simulink model "eovsa_corr_300mhz"  (R2012b)
settings: Solver=VariableStepDiscrete  SolverMode=SingleTasking  StartTime=0.0  StopTime=5000  RelTol=1e-3
undefined symbols (not defined in the file or in its folder): A, B, gcbh, PCIN, sfp, xlBlockLoadCallback, xlipgetpartsetting
libraries: xbsIndex_r4 x5996, casper_library_misc x52, simulink x33, dspsigops x24, xps_library x15, casper_library_delays x2
(part 26 of 65)

== system eovsa_corr_300mhz/vector_acc/power_sq_acc ==
  note: There is a bug in this green block.
      | Its output is held high for veector length number of pulses initially event without new_acc pulse.
  sync : Inport
  acc_length : Inport  Port=2
  sq_power_in0 : Inport  Port=3
  sq_power_in1 : Inport  Port=4
  sq_power_in2 : Inport  Port=5
  sq_power_in3 : Inport  Port=6
  sq_power_in4 : Inport  Port=7
  sq_power_in5 : Inport  Port=8
  sq_power_in6 : Inport  Port=9
  sq_power_in7 : Inport  Port=10
  acc_start_skip : Inport  Port=11
  Delay{1,3,6,9,14,17,21,24..40} (24 alike) : xbsIndex_r4/Delay  rst=off  infoeditControl=Selection of Reset will increase slice count due to use of real FFs and instead of SRLs  en=off  latency=1  dbl_ovrd=off  reg_retiming=on  block_type=delay
      settings: block_version=11.4
  Delay{2,4..5,7..8,10..13,15..16,18..20,22..23,41..42} (18 alike) : xbsIndex_r4/Delay  rst=off  infoeditControl=Selection of Reset will increase slice count due to use of real FFs and instead of SRLs  en=off  latency=1  dbl_ovrd=off  reg_retiming=off  block_type=delay
      settings: block_version=11.4
  Terminator{1..6,24} (7 alike) : Terminator
  new_acc1 : Subsystem
  wide_bram_vacc : Subsystem  AncestorBlock=casper_library_accumulators/wide_bram_vacc  mask(wide_bram_vacc){vec_len=2048, arith_type=Unsigned, n_bits=64, bin_pt=44}
      mask prompts: vec_len "Vector length:"; arith_type "Arithmetic type (input/output):"; n_bits "Bit width (output):"; bin_pt "Binary point (output):"
      mask help:
      | This vector accumulator based on DSP48 slices and BRAMs is designed for wide accumulators (48 < output width <= 96).
      |
      | It outputs its previous accumulated vector after a new_acc pulse is received.
      |
      | The "Data IN" (din) value is used if "Data OK" (dok) is 1, otherwise a 0 value is accumulated instead.  This can be used, for example, to implement blanking without requiring external multiplexers.
      mask init:
      | set_param([gcb,'/outsize/Reinterpret'], 'arith_type', arith_type);
      mask TypeOptions arith_type: Signed  (2's comp) | Unsigned
  wide_bram_vacc1 : Subsystem  AncestorBlock=casper_library_accumulators/wide_bram_vacc  mask(wide_bram_vacc){vec_len=2048, arith_type=Unsigned, n_bits=64, bin_pt=44}
      mask prompts: vec_len "Vector length:"; arith_type "Arithmetic type (input/output):"; n_bits "Bit width (output):"; bin_pt "Binary point (output):"
      mask help:
      | This vector accumulator based on DSP48 slices and BRAMs is designed for wide accumulators (48 < output width <= 96).
      |
      | It outputs its previous accumulated vector after a new_acc pulse is received.
      |
      | The "Data IN" (din) value is used if "Data OK" (dok) is 1, otherwise a 0 value is accumulated instead.  This can be used, for example, to implement blanking without requiring external multiplexers.
      mask init:
      | set_param([gcb,'/outsize/Reinterpret'], 'arith_type', arith_type);
      mask TypeOptions arith_type: Signed  (2's comp) | Unsigned
  wide_bram_vacc2 : Subsystem  AncestorBlock=casper_library_accumulators/wide_bram_vacc  mask(wide_bram_vacc){vec_len=2048, arith_type=Unsigned, n_bits=64, bin_pt=44}
      mask prompts: vec_len "Vector length:"; arith_type "Arithmetic type (input/output):"; n_bits "Bit width (output):"; bin_pt "Binary point (output):"
      mask help:
      | This vector accumulator based on DSP48 slices and BRAMs is designed for wide accumulators (48 < output width <= 96).
      |
      | It outputs its previous accumulated vector after a new_acc pulse is received.
      |
      | The "Data IN" (din) value is used if "Data OK" (dok) is 1, otherwise a 0 value is accumulated instead.  This can be used, for example, to implement blanking without requiring external multiplexers.
      mask init:
      | set_param([gcb,'/outsize/Reinterpret'], 'arith_type', arith_type);
      mask TypeOptions arith_type: Signed  (2's comp) | Unsigned
  wide_bram_vacc3 : Subsystem  AncestorBlock=casper_library_accumulators/wide_bram_vacc  mask(wide_bram_vacc){vec_len=2048, arith_type=Unsigned, n_bits=64, bin_pt=44}
      mask prompts: vec_len "Vector length:"; arith_type "Arithmetic type (input/output):"; n_bits "Bit width (output):"; bin_pt "Binary point (output):"
      mask help:
      | This vector accumulator based on DSP48 slices and BRAMs is designed for wide accumulators (48 < output width <= 96).
      |
      | It outputs its previous accumulated vector after a new_acc pulse is received.
      |
      | The "Data IN" (din) value is used if "Data OK" (dok) is 1, otherwise a 0 value is accumulated instead.  This can be used, for example, to implement blanking without requiring external multiplexers.
      mask init:
      | set_param([gcb,'/outsize/Reinterpret'], 'arith_type', arith_type);
      mask TypeOptions arith_type: Signed  (2's comp) | Unsigned
  wide_bram_vacc4 : Subsystem  AncestorBlock=casper_library_accumulators/wide_bram_vacc  mask(wide_bram_vacc){vec_len=2048, arith_type=Unsigned, n_bits=64, bin_pt=44}
      mask prompts: vec_len "Vector length:"; arith_type "Arithmetic type (input/output):"; n_bits "Bit width (output):"; bin_pt "Binary point (output):"
      mask help:
      | This vector accumulator based on DSP48 slices and BRAMs is designed for wide accumulators (48 < output width <= 96).
      |
      | It outputs its previous accumulated vector after a new_acc pulse is received.
      |
      | The "Data IN" (din) value is used if "Data OK" (dok) is 1, otherwise a 0 value is accumulated instead.  This can be used, for example, to implement blanking without requiring external multiplexers.
      mask init:
      | set_param([gcb,'/outsize/Reinterpret'], 'arith_type', arith_type);
      mask TypeOptions arith_type: Signed  (2's comp) | Unsigned
  wide_bram_vacc5 : Subsystem  AncestorBlock=casper_library_accumulators/wide_bram_vacc  mask(wide_bram_vacc){vec_len=2048, arith_type=Unsigned, n_bits=64, bin_pt=44}
      mask prompts: vec_len "Vector length:"; arith_type "Arithmetic type (input/output):"; n_bits "Bit width (output):"; bin_pt "Binary point (output):"
      mask help:
      | This vector accumulator based on DSP48 slices and BRAMs is designed for wide accumulators (48 < output width <= 96).
      |
      | It outputs its previous accumulated vector after a new_acc pulse is received.
      |
      | The "Data IN" (din) value is used if "Data OK" (dok) is 1, otherwise a 0 value is accumulated instead.  This can be used, for example, to implement blanking without requiring external multiplexers.
      mask init:
      | set_param([gcb,'/outsize/Reinterpret'], 'arith_type', arith_type);
      mask TypeOptions arith_type: Signed  (2's comp) | Unsigned
  wide_bram_vacc6 : Subsystem  AncestorBlock=casper_library_accumulators/wide_bram_vacc  mask(wide_bram_vacc){vec_len=2048, arith_type=Unsigned, n_bits=64, bin_pt=44}
      mask prompts: vec_len "Vector length:"; arith_type "Arithmetic type (input/output):"; n_bits "Bit width (output):"; bin_pt "Binary point (output):"
      mask help:
      | This vector accumulator based on DSP48 slices and BRAMs is designed for wide accumulators (48 < output width <= 96).
      |
      | It outputs its previous accumulated vector after a new_acc pulse is received.
      |
      | The "Data IN" (din) value is used if "Data OK" (dok) is 1, otherwise a 0 value is accumulated instead.  This can be used, for example, to implement blanking without requiring external multiplexers.
      mask init:
      | set_param([gcb,'/outsize/Reinterpret'], 'arith_type', arith_type);
      mask TypeOptions arith_type: Signed  (2's comp) | Unsigned
  wide_bram_vacc7 : Subsystem  AncestorBlock=casper_library_accumulators/wide_bram_vacc  mask(wide_bram_vacc){vec_len=2048, arith_type=Unsigned, n_bits=64, bin_pt=44}
      mask prompts: vec_len "Vector length:"; arith_type "Arithmetic type (input/output):"; n_bits "Bit width (output):"; bin_pt "Binary point (output):"
      mask help:
      | This vector accumulator based on DSP48 slices and BRAMs is designed for wide accumulators (48 < output width <= 96).
      |
      | It outputs its previous accumulated vector after a new_acc pulse is received.
      |
      | The "Data IN" (din) value is used if "Data OK" (dok) is 1, otherwise a 0 value is accumulated instead.  This can be used, for example, to implement blanking without requiring external multiplexers.
      mask init:
      | set_param([gcb,'/outsize/Reinterpret'], 'arith_type', arith_type);
      mask TypeOptions arith_type: Signed  (2's comp) | Unsigned
  data_valid : Outport
  power_sq0 : Outport  Port=2
  power_sq1 : Outport  Port=3
  power_sq2 : Outport  Port=4
  power_sq3 : Outport  Port=5
  power_sq4 : Outport  Port=6
  power_sq5 : Outport  Port=7
  power_sq6 : Outport  Port=8
  power_sq7 : Outport  Port=9
  wires:
  wide_bram_vacc/2(valid) -> data_valid/1
  wide_bram_vacc/1(dout) -> power_sq0/1
  wide_bram_vacc1/1(dout) -> power_sq1/1
  sync/1 -> new_acc1/1(sync)
  wide_bram_vacc1/2(valid) -> Terminator24/1
  wide_bram_vacc2/2(valid) -> Terminator1/1
  wide_bram_vacc2/1(dout) -> power_sq2/1
  wide_bram_vacc3/1(dout) -> power_sq3/1
  wide_bram_vacc4/2(valid) -> Terminator2/1
  wide_bram_vacc4/1(dout) -> power_sq4/1
  wide_bram_vacc5/2(valid) -> Terminator4/1
  wide_bram_vacc5/1(dout) -> power_sq5/1
  wide_bram_vacc6/1(dout) -> power_sq6/1
  wide_bram_vacc6/2(valid) -> Terminator6/1
  acc_length/1 -> new_acc1/2(acc_len)
  acc_start_skip/1 -> new_acc1/3(acc_start_skip)
  new_acc1/2(use_data) -> Delay41/1
  [use_data] -> Delay2/1
  new_acc1/1(new_acc) -> Delay42/1
  [new_acc] -> Delay19/1
  [use_data] -> Delay5/1
  [new_acc] -> Delay4/1
  [use_data] -> Delay8/1
  [new_acc] -> Delay7/1
  [use_data] -> Delay11/1
  [new_acc] -> Delay10/1
  [use_data] -> Delay13/1
  [new_acc] -> Delay12/1
  [use_data] -> Delay16/1
  [new_acc] -> Delay15/1
  [use_data] -> Delay20/1
  [new_acc] -> Delay18/1
  [use_data] -> Delay23/1
  [new_acc] -> Delay22/1
  sq_power_in0/1 -> Delay25/1
  sq_power_in1/1 -> Delay26/1
  sq_power_in2/1 -> Delay27/1
  sq_power_in3/1 -> Delay28/1
  sq_power_in4/1 -> Delay29/1
  sq_power_in5/1 -> Delay30/1
  sq_power_in7/1 -> Delay32/1
  sq_power_in6/1 -> Delay31/1
  Delay1/1 -> wide_bram_vacc/2(din)
  Delay2/1 -> wide_bram_vacc/3(dok)
  Delay19/1 -> wide_bram_vacc/1(new_acc)
  Delay3/1 -> wide_bram_vacc1/2(din)
  Delay4/1 -> wide_bram_vacc1/1(new_acc)
  Delay5/1 -> wide_bram_vacc1/3(dok)
  Delay6/1 -> wide_bram_vacc2/2(din)
  Delay7/1 -> wide_bram_vacc2/1(new_acc)
  Delay8/1 -> wide_bram_vacc2/3(dok)
  Delay10/1 -> wide_bram_vacc3/1(new_acc)
  Delay9/1 -> wide_bram_vacc3/2(din)
  Delay11/1 -> wide_bram_vacc3/3(dok)
  Delay14/1 -> wide_bram_vacc4/2(din)
  Delay13/1 -> wide_bram_vacc4/3(dok)
  Delay12/1 -> wide_bram_vacc4/1(new_acc)
  Delay16/1 -> wide_bram_vacc5/3(dok)
  Delay15/1 -> wide_bram_vacc5/1(new_acc)
  Delay17/1 -> wide_bram_vacc5/2(din)
  Delay18/1 -> wide_bram_vacc6/1(new_acc)
  Delay20/1 -> wide_bram_vacc6/3(dok)
  Delay21/1 -> wide_bram_vacc6/2(din)
  Delay25/1 -> Delay33/1
  Delay26/1 -> Delay34/1
  Delay27/1 -> Delay35/1
  Delay28/1 -> Delay36/1
  Delay29/1 -> Delay37/1
  Delay30/1 -> Delay38/1
  Delay31/1 -> Delay39/1
  Delay32/1 -> Delay40/1
  Delay33/1 -> Delay1/1
  Delay34/1 -> Delay3/1
  Delay35/1 -> Delay6/1
  Delay36/1 -> Delay9/1
  Delay37/1 -> Delay14/1
  Delay38/1 -> Delay17/1
  Delay39/1 -> Delay21/1
  Delay40/1 -> Delay24/1
  Delay41/1 -> [use_data]
  Delay42/1 -> [new_acc]
  wide_bram_vacc3/2(valid) -> Terminator3/1
  Delay23/1 -> wide_bram_vacc7/3(dok)
  Delay24/1 -> wide_bram_vacc7/2(din)
  Delay22/1 -> wide_bram_vacc7/1(new_acc)
  wide_bram_vacc7/1(dout) -> power_sq7/1
  wide_bram_vacc7/2(valid) -> Terminator5/1

== system eovsa_corr_300mhz/xeng0_vacc/edge_detect ==
  in : Inport
  Delay : xbsIndex_r4/Delay  rst=off  infoeditControl=Selection of Reset will increase slice count due to use of real FFs and instead of SRLs  en=off  latency=1  dbl_ovrd=off  reg_retiming=on  block_type=delay
      settings: xl_area=[0, 0, 0, 0, 0, 0, 0]
  Inverter : xbsIndex_r4/Inverter  en=off  latency=0  dbl_ovrd=off  block_type=inv
      settings: xl_area=[0, 0, 0, 0, 0, 0, 0]
  edge_op : xbsIndex_r4/Logical  logical_function=NOR  inputs=2  en=off  latency=0  precision=Full  arith_type=Unsigned  n_bits=8  bin_pt=2  align_bp=on  dbl_ovrd=off  block_type=logical
      settings: xl_area=[0, 0, 0, 0, 0, 0, 0]
  out : Outport
  wires:
  Inverter/1 -> edge_op/1
  edge_op/1 -> out/1
  in/1 -> Inverter/1, Delay/1
  Delay/1 -> edge_op/2

== system eovsa_corr_300mhz/xeng0_vacc/qv1 ==
  note: Compensate for the latency
      | of the vacc controller here.
      | (it sets rd_en high a clock
      | after vld goes high)
      | Then it takes a further clock to
      | mux and register the addr / enable signals
  rst : Inport
  rb_burst_len_mi : Inport  Port=2
  vld : Inport  Port=3
  sync : Inport  Port=4
  acc_len_mi : Inport  Port=5
  din : Inport  Port=6
  Constant : xbsIndex_r4/Constant  const="2^8 -  1"  gui_display_data_type=Fixed-point  arith_type=Unsigned  n_bits=8  bin_pt=0  preci_type=Single  exp_width=8  frac_width=24  explicit_period=on  period=1  equ=P=C  opselect=C  inp2=PCIN>>17  opr=+  inp1=P  carry=CIN  dbl_ovrd=off  block_type=constant
  Delay1 : xbsIndex_r4/Delay  rst=off  infoeditControl=Selection of Reset will increase slice count due to use of real FFs and instead of SRLs  en=off  latency=12-1  dbl_ovrd=off  reg_retiming=on  block_type=delay
  Delay2 : xbsIndex_r4/Delay  rst=off  infoeditControl=Selection of Reset will increase slice count due to use of real FFs and instead of SRLs  en=off  latency=2  dbl_ovrd=off  reg_retiming=on  block_type=delay
  Delay3 : xbsIndex_r4/Delay  rst=off  infoeditControl=Selection of Reset will increase slice count due to use of real FFs and instead of SRLs  en=off  latency=1  dbl_ovrd=off  reg_retiming=off  block_type=delay
  Delay4 : xbsIndex_r4/Delay  rst=off  infoeditControl=Selection of Reset will increase slice count due to use of real FFs and instead of SRLs  en=off  latency=2  dbl_ovrd=off  reg_retiming=off  block_type=delay
  Delay5 : xbsIndex_r4/Delay  rst=off  infoeditControl=Selection of Reset will increase slice count due to use of real FFs and instead of SRLs  en=off  latency=1  dbl_ovrd=off  reg_retiming=off  block_type=delay
  Delay6 : xbsIndex_r4/Delay  rst=off  infoeditControl=Selection of Reset will increase slice count due to use of real FFs and instead of SRLs  en=off  latency=12-1  dbl_ovrd=off  reg_retiming=on  block_type=delay
  Gateway Out{1..8} (8 alike) : xbsIndex_r4/Gateway Out  inherit_from_input=off  hdl_port=on  timing_constraint=None  locs_specified=off  LOCs={}  UseAsDAC=off  DACChannel='1'  block_type=gatewayout
  Inverter : xbsIndex_r4/Inverter  en=off  latency=0  dbl_ovrd=off  block_type=inv
  Inverter1 : xbsIndex_r4/Inverter  en=off  latency=0  dbl_ovrd=off  block_type=inv
  Logical : xbsIndex_r4/Logical  logical_function=AND  inputs=2  en=off  latency=0  precision=Full  arith_type=Unsigned  n_bits=16  bin_pt=0  align_bp=on  dbl_ovrd=off  block_type=logical
  Logical1 : xbsIndex_r4/Logical  logical_function=AND  inputs=2  en=off  latency=0  precision=Full  arith_type=Unsigned  n_bits=16  bin_pt=0  align_bp=on  dbl_ovrd=off  block_type=logical
  Scope : Scope  NumInputPorts=8
      settings: YMin=-5~-5~-5~-5~-5~-5~-5~-5  YMax=5~5~5~5~5~5~5~5
  Slice4 : xbsIndex_r4/Slice  nbits=64  boolean_output=off  mode=Lower Bit Location + Width  bit1=0  base1=MSB of Input  bit0=0  base0=LSB of Input  dbl_ovrd=off  block_type=slice
  Slice_A : xbsIndex_r4/Slice  nbits=32  boolean_output=off  mode=Lower Bit Location + Width  bit1=0  base1=MSB of Input  bit0=32  base0=LSB of Input  dbl_ovrd=off  block_type=slice
  Slice_A1 : xbsIndex_r4/Slice  nbits=32  boolean_output=off  mode=Lower Bit Location + Width  bit1=0  base1=MSB of Input  bit0=32  base0=LSB of Input  dbl_ovrd=off  block_type=slice
  Slice_A2 : xbsIndex_r4/Slice  nbits=32  boolean_output=off  mode=Lower Bit Location + Width  bit1=0  base1=MSB of Input  bit0=0  base0=LSB of Input  dbl_ovrd=off  block_type=slice
  Slice_A3 : xbsIndex_r4/Slice  nbits=32  boolean_output=off  mode=Lower Bit Location + Width  bit1=0  base1=MSB of Input  bit0=0  base0=LSB of Input  dbl_ovrd=off  block_type=slice
  adder1 : Subsystem
  adder2 : Subsystem
  bus_create : Subsystem  AncestorBlock=casper_library_flow_control/bus_create  mask(bus_create){inputNum=2}
      mask prompts: inputNum "Number of inputs:"
      mask init:
      | bus_create_init(gcb,...
      |     'inputNum', inputNum);
  pipeline1 : Subsystem  AncestorBlock=casper_library_delays/pipeline  mask(pipeline){latency=1}
      mask help:
      | An explicitly laid-out delay line to avoid mapping to SRL16s
      | for use in pipelining to help achieve timing closure.
      mask init:
      | pipeline_init(gcb,'latency',latency);
      settings: AttributesFormatString=Latency = %<latency>
      mask Display:
      | port_label('input', 1, 'd');
      | port_label('output', 1, 'q');
      | disp(['Z^-', num2str(latency)]);
  pipeline2 : Subsystem  AncestorBlock=casper_library_delays/pipeline  mask(pipeline){latency=1}
      mask help:
      | An explicitly laid-out delay line to avoid mapping to SRL16s
      | for use in pipelining to help achieve timing closure.
      mask init:
      | pipeline_init(gcb,'latency',latency);
      settings: AttributesFormatString=Latency = %<latency>
      mask Display:
      | port_label('input', 1, 'd');
      | port_label('output', 1, 'q');
      | disp(['Z^-', num2str(latency)]);
  pipeline3 : Subsystem  AncestorBlock=casper_library_delays/pipeline  mask(pipeline){latency=1}
      mask help:
      | An explicitly laid-out delay line to avoid mapping to SRL16s
      | for use in pipelining to help achieve timing closure.
      mask init:
      | pipeline_init(gcb,'latency',latency);
      settings: AttributesFormatString=Latency = %<latency>
      mask Display:
      | port_label('input', 1, 'd');
      | port_label('output', 1, 'q');
      | disp(['Z^-', num2str(latency)]);
  pipeline5 : Subsystem  AncestorBlock=casper_library_delays/pipeline  mask(pipeline){latency=1}
      mask help:
      | An explicitly laid-out delay line to avoid mapping to SRL16s
      | for use in pipelining to help achieve timing closure.
      mask init:
      | pipeline_init(gcb,'latency',latency);
      settings: AttributesFormatString=Latency = %<latency>
      mask Display:
      | port_label('input', 1, 'd');
      | port_label('output', 1, 'q');
      | disp(['Z^-', num2str(latency)]);
  pipeline6 : Subsystem  AncestorBlock=casper_library_delays/pipeline  mask(pipeline){latency=1}
      mask help:
      | An explicitly laid-out delay line to avoid mapping to SRL16s
      | for use in pipelining to help achieve timing closure.
      mask init:
      | pipeline_init(gcb,'latency',latency);
      settings: AttributesFormatString=Latency = %<latency>
      mask Display:
      | port_label('input', 1, 'd');
      | port_label('output', 1, 'q');
      | disp(['Z^-', num2str(latency)]);
  pipeline93 : Subsystem  AncestorBlock=casper_library_delays/pipeline  mask(pipeline){latency=1}
      mask help:
      | An explicitly laid-out delay line to avoid mapping to SRL16s
      | for use in pipelining to help achieve timing closure.
      mask init:
      | pipeline_init(gcb,'latency',latency);
      settings: AttributesFormatString=Latency = %<latency>
      mask Display:
      | port_label('input', 1, 'd');
      | port_label('output', 1, 'q');
      | disp(['Z^-', num2str(latency)]);
  qdr : xps_library/qdr  Tag=xps:qdr  which_qdr=qdr0  qdr_awidth=12  use_sniffer=on
  qdr_vacc_ctrl : Subsystem  mask{qdr_latency=12, add_latency=3, vec_len=vector_len}
      mask prompts: qdr_latency "QDR Latency?"; add_latency "Add latency?"; vec_len "Vector length?"
  dout : Outport
  dout_vld : Outport  Port=2
  first_vec : Outport  Port=3
  wires:
  Constant/1 -> qdr/3
  qdr/1 -> Slice4/1
  din/1 -> Delay2/1
  Delay1/1 -> pipeline1/1(d)
  [qdr_dout] -> Slice_A2/1  "adder_mem_in"
  pipeline1/1(q) -> Slice_A3/1  "adder_din"
  Slice4/1 -> pipeline5/1(d)
  [qdr_dout] -> dout/1  "vacc_dout"
  [rb_vld] -> dout_vld/1  "vacc_dvld"
  pipeline3/1(q) -> qdr/4  "adr_addr"
  Delay4/1 -> Delay5/1  "qdr_din"
  pipeline5/1(q) -> [qdr_dout]  "vacc_dout"
  bus_create/1(bus_out) -> Delay3/1
  Delay2/1 -> Delay6/1, Delay1/1
  [first_vec] -> adder1/3(new_acc)  "adder_first_vec"
  Delay3/1 -> Delay4/1
  [first_vec] -> first_vec/1
  rst/1 -> Gateway Out8/1, Inverter1/1, Inverter/1, qdr_vacc_ctrl/1(rst)  "rst"
  rb_burst_len_mi/1 -> Gateway Out1/1, qdr_vacc_ctrl/2(rb_burst_len_mi)  "burst length"
  vld/1 -> Gateway Out2/1, qdr_vacc_ctrl/3(vld)  "vld"
  sync/1 -> Gateway Out3/1, qdr_vacc_ctrl/4(sync)  "sync"
  acc_len_mi/1 -> Gateway Out7/1, qdr_vacc_ctrl/5(acc_len_mi)  "acc len"
  qdr_vacc_ctrl/1(qdr_re) -> Logical/2, Gateway Out4/1
  qdr_vacc_ctrl/2(qdr_we) -> Logical1/2, Gateway Out5/1
  qdr_vacc_ctrl/3(qdr_addr) -> Gateway Out6/1, pipeline3/1(d)
  qdr_vacc_ctrl/4(dout_vld) -> [rb_vld]
  qdr_vacc_ctrl/5(final_vec) -> [first_vec]
  Gateway Out2/1 -> Scope/3
  Gateway Out8/1 -> Scope/1
  Gateway Out7/1 -> Scope/5
  Gateway Out3/1 -> Scope/4
  Gateway Out6/1 -> Scope/8
  Gateway Out1/1 -> Scope/2
  Gateway Out5/1 -> Scope/7
  Gateway Out4/1 -> Scope/6
  Inverter/1 -> Logical/1
  pipeline2/1(q) -> qdr/2  "qdr_wr_en"
  pipeline93/1(q) -> qdr/1  "qdr_rd_en"
  Logical/1 -> pipeline93/1(d)
  Inverter1/1 -> Logical1/1
  Logical1/1 -> pipeline2/1(d)
  [first_vec] -> adder2/3(new_acc)
  Delay6/1 -> pipeline6/1(d)
  pipeline6/1(q) -> Slice_A1/1
  [qdr_dout] -> Slice_A/1
  Slice_A/1 -> adder2/1(buf_in)
  Slice_A1/1 -> adder2/2(din)
  Slice_A2/1 -> adder1/1(buf_in)
  Slice_A3/1 -> adder1/2(din)
  adder2/1(out) -> bus_create/1(in1)
  adder1/1(out) -> bus_create/2(in2)  "adder_dout"
  Delay5/1 -> qdr/5

== system eovsa_corr_300mhz/xeng_hdl_uint/xeng_descramble ==
  note: x_cast is necessary to correct for BRAM
      | readout order
  note: This bit of logic
      | ensures that we only send out
      | a sync if one was received
      | (and then align it with the start of a read)
  acc : Inport
  valid : Inport  Port=2
  sync : Inport  Port=3
  win_valid : Inport  Port=4
  Constant2 : xbsIndex_r4/Constant  const=0  gui_display_data_type=Fixed-point  arith_type=Boolean  n_bits=elements_bits + 1  bin_pt=0  preci_type=Single  exp_width=8  frac_width=24  explicit_period=on  period=1  equ=P=C  opselect=C  inp2=PCIN>>17  opr=+  inp1=P  carry=CIN  dbl_ovrd=off  block_type=constant
      settings: block_version=9.2.01
  Constant3 : xbsIndex_r4/Constant  const=0  gui_display_data_type=Fixed-point  arith_type=Unsigned  n_bits=n_bits_in/demux_factor  bin_pt=0  preci_type=Single  exp_width=8  frac_width=24  explicit_period=on  period=1  equ=P=C  opselect=C  inp2=PCIN>>17  opr=+  inp1=P  carry=CIN  dbl_ovrd=off  block_type=constant
      settings: block_version=9.2.01
  Delay1 : xbsIndex_r4/Delay  rst=off  infoeditControl=Selection of Reset will increase slice count due to use of real FFs and instead of SRLs  en=off  latency=3  dbl_ovrd=off  reg_retiming=off  block_type=delay
      settings: xl_area=[0, 0, 0, 0, 0, 0, 0]  block_version=9.2.01
  Delay{2..4,7} (4 alike) : xbsIndex_r4/Delay  rst=off  infoeditControl=Selection of Reset will increase slice count due to use of real FFs and instead of SRLs  en=off  latency=1  dbl_ovrd=off  reg_retiming=off  block_type=delay
      settings: xl_area=[0, 0, 0, 0, 0, 0, 0]  block_version=9.2.01
  Delay5 : xbsIndex_r4/Delay  rst=off  infoeditControl=Selection of Reset will increase slice count due to use of real FFs and instead of SRLs  en=off  latency=2  dbl_ovrd=off  reg_retiming=off  block_type=delay
      settings: xl_area=[0, 0, 0, 0, 0, 0, 0]  block_version=9.2.01
  Delay6 : xbsIndex_r4/Delay  rst=off  infoeditControl=Selection of Reset will increase slice count due to use of real FFs and instead of SRLs  en=off  latency=2  dbl_ovrd=off  reg_retiming=off  block_type=delay
      settings: xl_area=[0, 0, 0, 0, 0, 0, 0]  block_version=9.2.01
  Dual Port RAM : xbsIndex_r4/Dual Port RAM  depth=(num_elements+1)*demux_factor  initVector=[1:36*8]  distributed_mem=Block RAM  init_a=0  init_b=0  rst_a=off  rst_b=off  en_a=off  en_b=off  latency=3  write_mode_A=No Read On Write  write_mode_B=No Read On Write  dbl_ovrd=off  optimize=Speed  block_type=dpram
      settings: xl_area=[0, 0, 0, 0, 0, 0, 0]  block_version=9.2.01
  Gateway Out{4..11} (8 alike) : xbsIndex_r4/Gateway Out  inherit_from_input=off  hdl_port=off  timing_constraint=None  locs_specified=off  LOCs={}  UseAsDAC=off  DACChannel='1'  block_type=gatewayout
      settings: infoedit="Gateway out block.  Converts Xilinx fixed point inputs into ouputs of type Simulink integer, double, or fixed point.<P><P>Hardware notes:  In hardware these blocks become top level output ports or are discarded, depending on how they are configured."  xl_area=[0 0 0 0 0 0 0]  block_version=10.1.3
  Logical : xbsIndex_r4/Logical  logical_function=AND  inputs=2  en=off  latency=3  precision=Full  arith_type=Unsigned  n_bits=16  bin_pt=0  align_bp=on  dbl_ovrd=off  block_type=logical
  Register : xbsIndex_r4/Register  init=0  rst=on  en=on  dbl_ovrd=off  block_type=register
  Scope1 : Scope  NumInputPorts=8
      settings: TimeRange=70000  YMin=0~0~0~0~0~0~0~0  YMax=1~1~1~1~1~35~1~35  SaveName=ScopeData3
  Terminator1 : Terminator
  read_ctrl : Subsystem  AncestorBlock=casper_library_correlator/xeng_mask/win2_ctrl
  write_ctrl : Subsystem  AncestorBlock=casper_library_correlator/xeng_mask/win2_ctrl
  x_cast : Subsystem  AncestorBlock=casper_library_correlator/x_cast  mask{n_bits_in=n_bits_xeng_out, n_bits_out=n_bits_in/8, fix_pnt_pos=(n_bits-1)*2, demux_factor=demux_factor}
      mask prompts: n_bits_in "Number of bits (input)"; n_bits_out "Number of bits (output)"; fix_pnt_pos "Fixed point position"; demux_factor "Demux Factor"
      mask init:
      | switch (demux_factor)
      |     case (8)
      |         bit_offsets=[0 1 2 3 4 5 6 7];
      |     case (4) 
      |         bit_offsets=[1 0 3 2 5 4 7 6];  
      |     case (2) 
      |         bit_offsets=[3 2 1 0 7 6 5 4];  
      |     case (1) 
      |         bit_offsets=[7 6 5 4 3 2 1 0];  
      | end
      | 
      | 
      | fmtstr = sprintf('%d -> %d, demux %d.',n_bits_in,n_bits_out,demux_factor);
      | set_param(gcb, 'AttributesFormatString', fmtstr);
      settings: AttributesFormatString=18 -> 32, demux 4.
  acc_out : Outport
  valid_out : Outport  Port=2
  sync_out : Outport  Port=3
  wires:
  x_cast/1(out) -> Delay3/1
  Delay6/1 -> Gateway Out6/1
  Delay5/1 -> Gateway Out8/1
  [sync_in] -> Register/3
  [sync_in] -> Register/1
  [sync_in] -> Gateway Out5/1
  [valid_out] -> Gateway Out7/1
  [valid_out] -> Delay1/1
  read_ctrl/2(enable) -> [valid_out]
  [start_read] -> Gateway Out4/1
  [start_read] -> Register/2
  [start_read] -> Logical/1
  [start_read] -> read_ctrl/1(start)
  write_ctrl/1(start_readout) -> [start_read]
  win_valid/1 -> Delay5/1, write_ctrl/4(window_valid)
  Register/1 -> Logical/2
  Logical/1 -> sync_out/1
  Gateway Out10/1 -> Scope1/7
  Gateway Out9/1 -> Scope1/6
  Gateway Out7/1 -> Scope1/5
  Gateway Out4/1 -> Scope1/4
  Gateway Out5/1 -> Scope1/1
  Gateway Out6/1 -> Scope1/2
  Gateway Out8/1 -> Scope1/3
  Dual Port RAM/2 -> Terminator1/1
  acc/1 -> write_ctrl/2(data_in)
  write_ctrl/3(data_out) -> x_cast/1(in)
  Constant3/1 -> Dual Port RAM/2
  write_ctrl/4(enable) -> Delay2/1, Gateway Out10/1
  Constant2/1 -> Dual Port RAM/3
  Delay1/1 -> valid_out/1
  Dual Port RAM/1 -> acc_out/1
  read_ctrl/1(read_addr) -> Gateway Out9/1, Delay7/1
  write_ctrl/2(write_addr) -> Delay4/1, Gateway Out11/1
  sync/1 -> [sync_in], write_ctrl/1(sync)
  valid/1 -> Delay6/1, write_ctrl/3(xeng_valid)
  Gateway Out11/1 -> Scope1/8
  Delay2/1 -> Dual Port RAM/6
  Delay3/1 -> Dual Port RAM/5
  Delay4/1 -> Dual Port RAM/4
  Delay7/1 -> Dual Port RAM/1

== system eovsa_corr_300mhz/acc_sync/gen_N_pps/edge_detect2 ==
  in : Inport
  Delay : xbsIndex_r4/Delay  rst=off  infoeditControl=Selection of Reset will increase slice count due to use of real FFs and instead of SRLs  en=off  latency=1  dbl_ovrd=off  reg_retiming=on  block_type=delay
      settings: xl_area=[0, 0, 0, 0, 0, 0, 0]
  Inverter : xbsIndex_r4/Inverter  en=off  latency=0  dbl_ovrd=off  block_type=inv
      settings: xl_area=[0, 0, 0, 0, 0, 0, 0]
  edge_op : xbsIndex_r4/Logical  logical_function=AND  inputs=2  en=off  latency=0  precision=Full  arith_type=Unsigned  n_bits=8  bin_pt=2  align_bp=on  dbl_ovrd=off  block_type=logical
      settings: xl_area=[0, 0, 0, 0, 0, 0, 0]
  out : Outport
  wires:
  Inverter/1 -> edge_op/1
  edge_op/1 -> out/1
  in/1 -> Inverter/1, Delay/1
  Delay/1 -> edge_op/2

== system eovsa_corr_300mhz/adc/data_adc/add_gen ==
  note: To storage
  note: prevent one extra
      | write to address 0
  note: Do one
      | capture by
      | default
  note: Count of bytes in BRAM
      | as well as done signal
  note: A total count of
      | bytes written to
      | BRAM since trig
  note: Force MSbit of count
      | to be '1' by negating busy
      | as counter bit may be '0' or '1'
  vin : Inport
  din : Inport  Port=2
  we : Inport  Port=3
  go : Inport  Port=4
  cont : Inport  Port=5
  init : Inport  Port=6
  Concat : xbsIndex_r4/Concat  num_inputs=3  dbl_ovrd=off  block_type=concat
      settings: block_version=10.1.3
  Convert : xbsIndex_r4/Convert  gui_display_data_type=Fixed-point  arith_type=Unsigned  n_bits=32-nsamples-log2(increment)-1  bin_pt=0  float_type=Single  exp_bits=8  fraction_bits=24  quantization=Truncate  overflow=Wrap  en=off  latency=0  dbl_ovrd=off  pipeline=off  block_type=convert
      settings: block_version=10.1.3
  Delay{,1..7} (8 alike) : xbsIndex_r4/Delay  rst=off  infoeditControl=Selection of Reset will increase slice count due to use of real FFs and instead of SRLs  en=off  latency=1  dbl_ovrd=off  reg_retiming=on  block_type=delay
      settings: block_version=11.4
  Inverter : xbsIndex_r4/Inverter  en=off  latency=1  dbl_ovrd=off  block_type=inv
      settings: block_version=11.4
  Inverter1 : xbsIndex_r4/Inverter  en=off  latency=0  dbl_ovrd=off  block_type=inv
      settings: block_version=11.4
  Logical1 : xbsIndex_r4/Logical  logical_function=AND  inputs=2  en=off  latency=1  precision=Full  arith_type=Unsigned  n_bits=8  bin_pt=2  align_bp=on  dbl_ovrd=off  block_type=logical
      settings: xl_area=[0, 0, 0, 0, 0, 0, 0]
  Logical2 : xbsIndex_r4/Logical  logical_function=AND  inputs=2  en=off  latency=1  precision=Full  arith_type=Unsigned  n_bits=8  bin_pt=2  align_bp=on  dbl_ovrd=off  block_type=logical
      settings: xl_area=[0, 0, 0, 0, 0, 0, 0]
  Logical4 : xbsIndex_r4/Logical  logical_function=OR  inputs=2  en=off  latency=0  precision=Full  arith_type=Unsigned  n_bits=8  bin_pt=2  align_bp=on  dbl_ovrd=off  block_type=logical
      settings: xl_area=[0, 0, 0, 0, 0, 0, 0]
  Logical6 : xbsIndex_r4/Logical  logical_function=AND  inputs=3  en=off  latency=0  precision=Full  arith_type=Unsigned  n_bits=8  bin_pt=2  align_bp=on  dbl_ovrd=off  block_type=logical
      settings: xl_area=[0, 0, 0, 0, 0, 0, 0]
  Register3 : xbsIndex_r4/Register  init=0  rst=on  en=on  dbl_ovrd=off  block_type=register
      settings: xl_area=[0, 0, 0, 0, 0, 0, 0]
  Register4 : xbsIndex_r4/Register  init=0  rst=off  en=on  dbl_ovrd=off  block_type=register
      settings: xl_area=[0, 0, 0, 0, 0, 0, 0]
  Register5 : xbsIndex_r4/Register  init=1  rst=on  en=on  dbl_ovrd=off  block_type=register
      settings: xl_area=[0, 0, 0, 0, 0, 0, 0]
  Shift : xbsIndex_r4/Shift  shift_dir=Left  shift_bits=32-nsamples-log2(increment)-1-1  en=off  latency=1  precision=Full  arith_type="Signed  (2's comp)"  n_bits=16  bin_pt=14  quantization=Truncate  overflow=Wrap  dbl_ovrd=off  block_type=shift
  add_gen : xbsIndex_r4/Counter  cnt_type=Free Running  cnt_to=1  operation=Up  start_count=0  cnt_by_val=increment  arith_type=Unsigned  n_bits=counter_size  bin_pt=0  load_pin=off  rst=on  en=on  explicit_period=on  period=1  dbl_ovrd=off  use_behavioral_HDL=off  implementation=DSP48  use_rpm=on  block_type=counter
      settings: xl_area=[0, 0, 0, 0, 0, 0, 0]
  edge_detect : Subsystem  AncestorBlock=casper_library_misc/edge_detect  mask(edge_detect){edge=Both, polarity=Active High, x_in=[0 0.08 0.08 0.16 0.16 0.24 0.24 0.32 0.32 0.4], y_in=[-1 -1  1  1  1  1 -1 -1 -1 -1], x_out=[0.6 0.68 0.68 0.76 0.76 0.84 0.84 0.92 0.92 1], y_out=[-1 -1  1  1 -1 -1  1  1 -1 -1]}
      mask prompts: edge "Edge Type"; polarity "Output Polarity"; x_in "Input X Positions"; y_in "Input Y Positions"; x_out "Output X Positions"; y_out "Output Y Positions"
      mask help: Output is active for one-cycle after each edge of the specified type (i.e. rising, falling or both).
      mask init: same as eovsa_corr_300mhz/edge_detect1
      settings: AttributesFormatString=|
      | both edges
      | active high
      mask Help: Output is active for one-cycle after each edge of the specified type (i.e. rising, falling, or both).  Latency is zero.
      mask TypeOptions edge: Rising | Falling | Both
      mask TypeOptions polarity: Active High | Active Low
      mask Display:
      | plot(x_in_num,0.5+y_in_num*0.2);
      | plot(x_out_num,0.5+y_out_num*0.2);
  slice1 : xbsIndex_r4/Slice  nbits=nsamples+log2(increment)  boolean_output=off  mode=Lower Bit Location + Width  bit1=0  base1=LSB of Input  bit0=0  base0=LSB of Input  dbl_ovrd=off  block_type=slice
      settings: block_version=10.1.3
  slice2 : xbsIndex_r4/Slice  nbits=nsamples-burst_size  boolean_output=off  mode=Lower Bit Location + Width  bit1=0  base1=LSB of Input  bit0=log2(increment)+burst_size  base0=LSB of Input  dbl_ovrd=off  block_type=slice
      settings: block_version=10.1.3
  slice3 : xbsIndex_r4/Slice  nbits=1  boolean_output=on  mode=Lower Bit Location + Width  bit1=0  base1=MSB of Input  bit0=nsamples + log2(increment)  base0=LSB of Input  dbl_ovrd=off  block_type=slice
      settings: block_version=10.1.3
  vout : Outport
  add : Outport  Port=2
  dout : Outport  Port=3
  we_o : Outport  Port=4
  status : Outport  Port=5
  en_cnt : Outport  Port=6
  wires:
  Shift/1 -> Concat/1
  Delay/1 -> Register5/2
  Inverter1/1 -> Logical4/2
  cont/1 -> Delay3/1
  edge_detect/1(out) -> Inverter1/1, Register5/3
  Register4/1 -> vout/1
  Logical2/1 -> Register4/2
  Register3/1 -> Logical2/2
  vin/1 -> Delay5/1
  add_gen/1 -> slice2/1, slice1/1, Delay2/1, slice3/1
  Register5/1 -> Convert/1, Inverter/1, Logical6/1
  slice3/1 -> edge_detect/1(in)
  init/1 -> Delay4/1
  Logical6/1 -> we_o/1, Logical2/1, Register3/2, add_gen/2
  Concat/1 -> status/1
  Convert/1 -> Shift/1
  slice2/1 -> add/1
  Delay2/1 -> en_cnt/1
  din/1 -> Delay6/1
  Delay1/1 -> Concat/3
  slice1/1 -> Delay1/1
  Inverter/1 -> Concat/2
  Logical4/1 -> Logical6/2
  we/1 -> Logical1/1
  go/1 -> Logical1/2
  Logical1/1 -> Logical6/3
  Delay7/1 -> Register4/1
  Delay3/1 -> Logical4/1, Register5/1
  Delay4/1 -> Register3/3, Register3/1, add_gen/1, Delay/1
  Delay5/1 -> Delay7/1
  Delay6/1 -> dout/1

== system eovsa_corr_300mhz/adc/data_adc/basic_ctrl ==
  vin : Inport
  din : Inport  Port=2
  we : Inport  Port=3
  trig : Inport  Port=4
  ctrl : Inport  Port=5
  stopi : Inport  Port=6
  Constant : xbsIndex_r4/Constant  const=1  gui_display_data_type=Fixed-point  arith_type=Boolean  n_bits=16  bin_pt=14  preci_type=Single  exp_width=8  frac_width=24  explicit_period=on  period=1  equ=P=C  opselect=C  inp2=PCIN>>17  opr=+  inp1=P  carry=CIN  dbl_ovrd=off  block_type=constant
      settings: block_version=11.4
  Constant1 : xbsIndex_r4/Constant  const=1  gui_display_data_type=Fixed-point  arith_type=Boolean  n_bits=1  bin_pt=0  preci_type=Single  exp_width=8  frac_width=24  explicit_period=on  period=1  equ=P=C  opselect=C  inp2=PCIN>>17  opr=+  inp1=P  carry=CIN  dbl_ovrd=off  block_type=constant
  Constant2 : xbsIndex_r4/Constant  const=1  gui_display_data_type=Fixed-point  arith_type=Boolean  n_bits=1  bin_pt=0  preci_type=Single  exp_width=8  frac_width=24  explicit_period=on  period=1  equ=P=C  opselect=C  inp2=PCIN>>17  opr=+  inp1=P  carry=CIN  dbl_ovrd=off  block_type=constant
  Delay1 : xbsIndex_r4/Delay  rst=off  infoeditControl=Selection of Reset will increase slice count due to use of real FFs and instead of SRLs  en=off  latency=1  dbl_ovrd=off  reg_retiming=on  block_type=delay
      settings: block_version=11.4
  Delay2 : xbsIndex_r4/Delay  rst=off  infoeditControl=Selection of Reset will increase slice count due to use of real FFs and instead of SRLs  en=off  latency=1  dbl_ovrd=off  reg_retiming=on  block_type=delay
      settings: block_version=11.4
  Delay3 : xbsIndex_r4/Delay  rst=off  infoeditControl=Selection of Reset will increase slice count due to use of real FFs and instead of SRLs  en=off  latency=1  dbl_ovrd=off  reg_retiming=on  block_type=delay
      settings: block_version=11.4
  Inverter : xbsIndex_r4/Inverter  en=off  latency=0  dbl_ovrd=off  block_type=inv
      settings: block_version=11.4
  Logical : xbsIndex_r4/Logical  logical_function=AND  inputs=2  en=off  latency=0  precision=Full  arith_type=Unsigned  n_bits=16  bin_pt=0  align_bp=on  dbl_ovrd=off  block_type=logical
      settings: block_version=11.4
  Mux1 : xbsIndex_r4/Mux  inputs=2  en=off  latency=0  precision=Full  arith_type="Signed  (2's comp)"  n_bits=8  bin_pt=2  quantization=Truncate  overflow=Wrap  dbl_ovrd=off  block_type=mux
      settings: xl_area=[0, 0, 0, 0, 0, 0, 0]
  Mux2 : xbsIndex_r4/Mux  inputs=2  en=off  latency=0  precision=Full  arith_type="Signed  (2's comp)"  n_bits=8  bin_pt=2  quantization=Truncate  overflow=Wrap  dbl_ovrd=off  block_type=mux
      settings: xl_area=[0, 0, 0, 0, 0, 0, 0]
  Register1 : xbsIndex_r4/Register  init=0  rst=on  en=on  dbl_ovrd=off  block_type=register
      settings: xl_area=[0, 0, 0, 0, 0, 0, 0]
  Register6 : xbsIndex_r4/Register  init=0  rst=on  en=on  dbl_ovrd=off  block_type=register
      settings: xl_area=[0, 0, 0, 0, 0, 0, 0]
  dram_munge : Subsystem  mask{dram=off, data_width=data_width}
      mask prompts: data_width "data width"
      mask init: same as eovsa_corr_300mhz/rx_hdr/basic_ctrl/dram_munge
  edge_detect : casper_library_misc/edge_detect  edge=Rising  polarity=Active High  x_in=[0 0.08 0.08 0.16 0.16 0.24 0.24 0.32 0.32 0.4]  y_in="[-1 -1  1  1  1  1  1  1  1  1]"  x_out=[0.6 0.68 0.68 0.76 0.76 0.84 0.84 0.92 0.92 1]  y_out="[-1 -1  1  1 -1 -1 -1 -1 -1 -1]"
  enable : xbsIndex_r4/Slice  nbits=1  boolean_output=on  mode=Lower Bit Location + Width  bit1=0  base1=LSB of Input  bit0=0  base0=LSB of Input  dbl_ovrd=off  block_type=slice
      settings: infoedit="Extracts a given range of bits from each input sample and presents it at the output.  The output type is ordinarily unsigned with binary point at zero, but can be Boolean when the slice is one bit wide.<P><P>Hardware notes: In hardware this block costs nothing."  block_version=10.1.3
  trig_src : xbsIndex_r4/Slice  nbits=1  boolean_output=on  mode=Lower Bit Location + Width  bit1=0  base1=LSB of Input  bit0=1  base0=LSB of Input  dbl_ovrd=off  block_type=slice
      settings: infoedit="Extracts a given range of bits from each input sample and presents it at the output.  The output type is ordinarily unsigned with binary point at zero, but can be Boolean when the slice is one bit wide.<P><P>Hardware notes: In hardware this block costs nothing."  block_version=10.1.3
  valid_src : xbsIndex_r4/Slice  nbits=1  boolean_output=on  mode=Lower Bit Location + Width  bit1=0  base1=LSB of Input  bit0=2  base0=LSB of Input  dbl_ovrd=off  block_type=slice
      settings: infoedit="Extracts a given range of bits from each input sample and presents it at the output.  The output type is ordinarily unsigned with binary point at zero, but can be Boolean when the slice is one bit wide.<P><P>Hardware notes: In hardware this block costs nothing."  block_version=10.1.3
  vout : Outport
  dout : Outport  Port=2
  we_o : Outport  Port=3
  go : Outport  Port=4
  stop : Outport  Port=5
  init : Outport  Port=6
  wires:
  Delay1/1 -> edge_detect/1
  Delay3/1 -> Mux1/1
  Delay2/1 -> Mux2/1
  dram_munge/1(vout) -> vout/1
  vin/1 -> dram_munge/1(vin)
  dram_munge/3(we_o) -> we_o/1
  dram_munge/2(dout) -> dout/1
  din/1 -> dram_munge/2(din)
  Inverter/1 -> Logical/2
  Mux2/1 -> Logical/1, Register6/1
  Register6/1 -> go/1
  trig/1 -> Mux2/2
  Mux1/1 -> dram_munge/3(we)
  we/1 -> Mux1/2
  ctrl/1 -> enable/1, valid_src/1, trig_src/1
  edge_detect/1 -> Inverter/1, Register1/3, dram_munge/4(init), Register6/2, init/1
  enable/1 -> Delay1/1
  Constant1/1 -> Mux2/3
  Constant2/1 -> Mux1/3
  trig_src/1 -> Delay2/1
  valid_src/1 -> Delay3/1
  Constant/1 -> Register1/1
  Register1/1 -> Register6/3
  Logical/1 -> Register1/2
  stopi/1 -> stop/1

== system eovsa_corr_300mhz/adc/data_adc/bram ==
  addr : Inport
  data_in : Inport  Port=2
  we : Inport  Port=3
  calc_add : Subsystem  mask{data_width=32, addr_width=11, sample_rate=sample_rate}
      mask prompts: data_width "data width"; addr_width "address width"; sample_rate "sample rate"
  convert_addr : xbsIndex_r4/Convert  gui_display_data_type=Fixed-point  arith_type=Unsigned  n_bits=addr_width  bin_pt=0  float_type=Single  exp_bits=8  fraction_bits=24  quantization=Truncate  overflow=Wrap  en=off  latency=0  dbl_ovrd=off  pipeline=off  block_type=convert
      settings: xl_area=[0, 0, 0, 0, 0, 0, 0]
  convert_din1 : xbsIndex_r4/Convert  gui_display_data_type=Fixed-point  arith_type=Unsigned  n_bits=32  bin_pt=0  float_type=Single  exp_bits=8  fraction_bits=24  quantization=Truncate  overflow=Wrap  en=off  latency=0  dbl_ovrd=off  pipeline=off  block_type=convert
      settings: xl_area=[0, 0, 0, 0, 0, 0, 0]
  convert_we : xbsIndex_r4/Convert  gui_display_data_type=Fixed-point  arith_type=Unsigned  n_bits=1  bin_pt=0  float_type=Single  exp_bits=8  fraction_bits=24  quantization=Truncate  overflow=Wrap  en=off  latency=0  dbl_ovrd=off  pipeline=off  block_type=convert
      settings: xl_area=[0, 0, 0, 0, 0, 0, 0]
  eovsa_corr_300mhz_adc_data_adc_bram_addr : xbsIndex_r4/Gateway Out  inherit_from_input=off  hdl_port=on  timing_constraint=None  locs_specified=off  LOCs={'A5','B9','A9','C1','A3','G6','E9','A6','A7','A8','B8','B1','B3','D9','B5','B4','B6','C2'}  UseAsDAC=off  DACChannel='1'  block_type=gatewayout
      settings: infoedit="Gateway out block.  Converts Xilinx fixed point inputs into ouputs of type Simulink integer, double, or fixed point.<P><P>Hardware notes:  In hardware these blocks become top level output ports or are discarded, depending on how they are configured."  xl_area=[0, 0, 0, 0, 0, 0, 0]  sginterface={'Nallatech'=>{'xdspkit'=>{'non_memory_mapped_port'=>'uprev_Shared_BRAM_addr'}},'Xilinx'=>{'jtaghwcosim'=>{'non_memory_mapped_port'=>'uprev_Shared_BRAM_addr'},'xdspkit'=>{'non_memory_mapped_port'=>'uprev_Shared_BRAM_addr'}}}
  eovsa_corr_300mhz_adc_data_adc_bram_data_in : xbsIndex_r4/Gateway Out  inherit_from_input=off  hdl_port=on  timing_constraint=None  locs_specified=off  LOCs={'B21','B22','A22','B23','B19','C19','A20','A21','A23','B24','A24','A25','E18','D18','C18','B18'}  UseAsDAC=off  DACChannel='1'  block_type=gatewayout
      settings: infoedit="Gateway out block.  Converts Xilinx fixed point inputs into ouputs of type Simulink integer, double, or fixed point.<P><P>Hardware notes:  In hardware these blocks become top level output ports or are discarded, depending on how they are configured."  xl_area=[0, 0, 0, 0, 0, 0, 0]  sginterface={'Nallatech'=>{'xdspkit'=>{'non_memory_mapped_port'=>'uprev_Shared_BRAM_data_in'}},'Xilinx'=>{'jtaghwcosim'=>{'non_memory_mapped_port'=>'uprev_Shared_BRAM_data_in'},'xdspkit'=>{'non_memory_mapped_port'=>'uprev_Shared_BRAM_data_in'}}}
  eovsa_corr_300mhz_adc_data_adc_bram_data_out : xbsIndex_r4/Gateway In  gui_display_data_type=Fixed-point  arith_type=Unsigned  n_bits=32  bin_pt=0  preci_type=Single  exp_width=8  frac_width=24  quantization=Truncate  overflow=Wrap  period=sample_rate  dbl_ovrd=off  timing_constraint=None  locs_specified=off  LOCs={}  UseAsADC=off  ADCChannel='1'  inherit_from_input=off  hdl_port=on  block_type=gatewayin
      settings: xl_area=[0, 0, 0, 0, 0, 0, 0]
  eovsa_corr_300mhz_adc_data_adc_bram_we : xbsIndex_r4/Gateway Out  inherit_from_input=off  hdl_port=on  timing_constraint=None  locs_specified=off  LOCs={'A14'}  UseAsDAC=off  DACChannel='1'  block_type=gatewayout
      settings: infoedit="Gateway out block.  Converts Xilinx fixed point inputs into ouputs of type Simulink integer, double, or fixed point.<P><P>Hardware notes:  In hardware these blocks become top level output ports or are discarded, depending on how they are configured."  xl_area=[0, 0, 0, 0, 0, 0, 0]
  mem : Subsystem
  munge_in : Subsystem  AncestorBlock=casper_library_flow_control/munge  mask(munge){divisions=1, div_size=32, order=[0], arith_type_out=Unsigned, bin_pt_out=0}
      mask prompts: divisions "Number of divisions"; div_size "Division size (bits)"; order "Division packing order"; arith_type_out "Output arithmetic type"; bin_pt_out "Output binary point"
      mask help: Splits an input bus into the specified number of divisions and then recombines them in the order specified (most significant division = 0,least = number divisions-1)
      mask init:
      | munge_init(gcb, ...
      |     'divisions', divisions, ...
      |     'div_size', div_size, ...
      |     'order', order, ...
      |     'arith_type_out', arith_type_out, ...
      |     'bin_pt_out', bin_pt_out);
      settings: AttributesFormatString=|
      | split:32
      | join:0
      | Unsigned [32,0]
      mask TypeOptions arith_type_out: Unsigned | Signed  (2's comp) | Floating-point
  munge_out : Subsystem  AncestorBlock=casper_library_flow_control/munge  mask(munge){divisions=1, div_size=32, order=[0], arith_type_out=Unsigned, bin_pt_out=0}
      mask prompts: divisions "Number of divisions"; div_size "Division size (bits)"; order "Division packing order"; arith_type_out "Output arithmetic type"; bin_pt_out "Output binary point"
      mask help: Splits an input bus into the specified number of divisions and then recombines them in the order specified (most significant division = 0,least = number divisions-1)
      mask init:
      | munge_init(gcb, ...
      |     'divisions', divisions, ...
      |     'div_size', div_size, ...
      |     'order', order, ...
      |     'arith_type_out', arith_type_out, ...
      |     'bin_pt_out', bin_pt_out);
      settings: AttributesFormatString=|
      | split:32
      | join:0
      | Unsigned [32,0]
      mask TypeOptions arith_type_out: Unsigned | Signed  (2's comp) | Floating-point
  data_out : Outport
  wires:
  munge_in/1(dout) -> convert_din1/1
  munge_out/1(dout) -> data_out/1
  we/1 -> convert_we/1
  addr/1 -> calc_add/1(in)
  mem/1(Out1) -> eovsa_corr_300mhz_adc_data_adc_bram_data_out/1
  eovsa_corr_300mhz_adc_data_adc_bram_data_out/1 -> munge_out/1(din)
  convert_we/1 -> eovsa_corr_300mhz_adc_data_adc_bram_we/1
  eovsa_corr_300mhz_adc_data_adc_bram_addr/1 -> mem/1(In1)
  eovsa_corr_300mhz_adc_data_adc_bram_data_in/1 -> mem/2(In2)
  eovsa_corr_300mhz_adc_data_adc_bram_we/1 -> mem/3(In3)
  calc_add/1(out) -> convert_addr/1
  data_in/1 -> munge_in/1(din)
  convert_din1/1 -> eovsa_corr_300mhz_adc_data_adc_bram_data_in/1
  convert_addr/1 -> eovsa_corr_300mhz_adc_data_adc_bram_addr/1

== system eovsa_corr_300mhz/adc/data_adc/ctrl ==
  sim_1 : Inport
  eovsa_corr_300mhz_adc_data_adc_ctrl_user_data_out : xbsIndex_r4/Gateway In  gui_display_data_type=Fixed-point  arith_type=Unsigned  n_bits=32  bin_pt=0  preci_type=Single  exp_width=8  frac_width=24  quantization="Round  (unbiased: +/- Inf)"  overflow=Saturate  period=1  dbl_ovrd=off  timing_constraint=None  locs_specified=off  LOCs={}  UseAsADC=off  ADCChannel='1'  inherit_from_input=off  hdl_port=on  block_type=gatewayin
  io_delay : xbsIndex_r4/Delay  rst=off  infoeditControl=Selection of Reset will increase slice count due to use of real FFs and instead of SRLs  en=off  latency=0  dbl_ovrd=off  reg_retiming=on  block_type=delay
  reint1 : xbsIndex_r4/Reinterpret  force_arith_type=on  arith_type=Unsigned  force_bin_pt=on  bin_pt=0  block_type=reinterpret
  slice_reg : xbsIndex_r4/Slice  nbits=32  boolean_output=off  mode=Lower Bit Location + Width  bit1=0  base1=MSB of Input  bit0=0  base0=LSB of Input  dbl_ovrd=off  block_type=slice
  in_reg : Outport
  wires:
  eovsa_corr_300mhz_adc_data_adc_ctrl_user_data_out/1 -> io_delay/1
  sim_1/1 -> eovsa_corr_300mhz_adc_data_adc_ctrl_user_data_out/1
  io_delay/1 -> slice_reg/1
  slice_reg/1 -> reint1/1
  reint1/1 -> in_reg/1
